simulink library "visionmorphops"  (R2015b)
settings: Solver=ode45  SolverMode=SingleTasking  StartTime=0.0  StopTime=10.0  RelTol=1e-3
undefined symbols (not defined in the file or in its folder): nhdims, nhood
undefined symbols (not defined in the file): strel
libraries: visionmorphops x2
settings Model: ExtModeAutoUpdateStatusClock=off  Creator=The MathWorks, Inc.  LastModifiedBy=The MathWorks, Inc.
settings DataIOCC: SaveFormat=Array  SignalLoggingSaveFormat=ModelDataLogs
settings OptimizationCC: BlockReduction=off  BooleanDataType=off
settings DebuggingCC: SaveWithParameterizedLinksMsg=none  UnderspecifiedInitializationDetection=Classic  MergeDetectMultiDrivingBlocksExec=none  SignalResolutionControl=TryResolveAllWithWarning  StrictBusMsg=Warning
settings HardwareCC: ProdBitPerPointer=32  ProdLargestAtomicFloat=None  ProdIntDivRoundTo=Undefined  ProdEndianess=Unspecified  ProdWordSize=32  ProdHWDeviceType=32-bit Generic  TargetUnknown=on
settings SFSimCC: SimGenImportedTypeDefs=on
settings GRTTargetCC: GeneratePreprocessorConditionals=Disable all
settings ConfigComp: CovModelRefEnable=Off

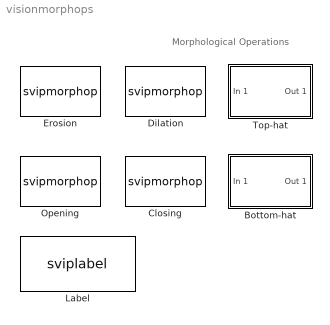
== system visionmorphops ==
  note: Morphological Operations
  Bottom-hat : Subsystem  mask(Bottom-hat){imgtype=Intensity, nhoodsrc=Specify via dialog, strel=strel('octagon',15)}
      mask prompts: imgtype "Input image type:"; nhoodsrc "Neighborhood or structuring element source:"; strel "Neighborhood or structuring element:"
      mask help:
      | Perform morphological bottom-hat filtering on an intensity or binary image.
      |
      | Use the Neighborhood or structuring element parameter to define the neighborhood or structuring element that the block applies to the image.  Specify a neighborhood by entering a matrix or vector of ones and zeros.  Specify a structuring element using the strel function.  Alternatively, you can specify neighborhood values using the Nhood port.
      |
      | For further information on structuring elements, type doc strel at the MATLAB command prompt.
      mask init:
      | nhoodsrc_str = get_param(gcbh,'nhoodsrc');
      | imgtype_str  = get_param(gcbh,'imgtype');
      | if strncmp(nhoodsrc_str,'Specify',5)
      | 	[si(1:2).port] = deal(1,1);
      | 	[si(1:2).txt] = deal('','');
      | else
      | 	[si(1:2).port] = deal(1,2);
      | 	if strncmp(imgtype_str,'Bina',4)
      | 		[si(1:2).txt] = deal('BW','Nhood');
      | 	else
      | 		[si(1:2).txt] = deal('I','Nhood');
      | 	end
      | end
      | 
      | vipblkhatfilter('init')
      mask Help: eval('visionblockhelp');
      mask TypeOptions imgtype: Intensity | Binary
      mask TypeOptions nhoodsrc: Specify via dialog | Input port
      mask Callback nhoodsrc: vipblkhatfilter
      mask Display:
      | disp('Bottom-hat')
      | port_label('input',si(1).port, si(1).txt);
      | port_label('input',si(2).port, si(2).txt);
  Closing : S-Function  FunctionName=svipmorphop  Parameters=3,nhoodsrc,nhood,nhdims  SFunctionDeploymentMode=off  EnableBusSupport=on  mask(Closing){nhoodsrc=Specify via dialog, strel=strel('line',5,45)}
      mask prompts: nhoodsrc "Neighborhood or structuring element source:"; strel "Neighborhood or structuring element:"
      mask help:
      | Perform morphological closing on an intensity or binary image.
      |
      | Use the Neighborhood or structuring element parameter to define the neighborhood or structuring element that the block applies to the image.  Specify a neighborhood by entering a matrix or vector of ones and zeros.  Specify a structuring element using the strel function.  Alternatively, you can specify neighborhood values using the Nhood port.
      |
      | For further information on structuring elements, type doc strel at the MATLAB command prompt.
      mask init:
      | nhoodsrc_str = get_param(gcbh,'nhoodsrc');
      | if strncmp(nhoodsrc_str,'Specify',5)
      | 	[si(1:2).port] = deal(1,1);
      | 	[si(1:2).txt] = deal('','');
      | else
      | 	[si(1:2).port] = deal(1,2);
      | 	[si(1:2).txt] = deal('I','Nhood');
      | end
      | [nhood nhdims] = vipblkmorphop(strel);
      mask Help: eval('visionblockhelp');
      mask TypeOptions nhoodsrc: Specify via dialog | Input port
      mask Callback nhoodsrc: vipblkmorphop
      mask Display:
      | disp('Close');
      | port_label('input',si(1).port, si(1).txt);
      | port_label('input',si(2).port, si(2).txt);
  Dilation : S-Function  FunctionName=svipmorphop  Parameters=1,nhoodsrc,nhood,nhdims  SFunctionDeploymentMode=off  EnableBusSupport=on  mask(Dilation){nhoodsrc=Specify via dialog, strel=[1 1; 1 1]}
      mask prompts: nhoodsrc "Neighborhood or structuring element source:"; strel "Neighborhood or structuring element:"
      mask help:
      | Perform morphological dilation on an intensity or binary image.
      |
      | Use the Neighborhood or structuring element parameter to define the neighborhood or structuring element that the block applies to the image.  Specify a neighborhood by entering a matrix or vector of ones and zeros.  Specify a structuring element using the strel function.  Alternatively, you can specify neighborhood values using the Nhood port.
      |
      | For further information on structuring elements, type doc strel at the MATLAB command prompt.
      mask init: same as visionmorphops/Closing
      mask Help: eval('visionblockhelp');
      mask TypeOptions nhoodsrc: Specify via dialog | Input port
      mask Callback nhoodsrc: vipblkmorphop
      mask Display:
      | disp('Dilate');
      | port_label('input',si(1).port, si(1).txt);
      | port_label('input',si(2).port, si(2).txt);
  Erosion : S-Function  FunctionName=svipmorphop  Parameters=0,nhoodsrc,nhood,nhdims  SFunctionDeploymentMode=off  EnableBusSupport=on  mask(Erosion){nhoodsrc=Specify via dialog, strel=strel('square',4)}
      mask prompts: nhoodsrc "Neighborhood or structuring element source:"; strel "Neighborhood or structuring element:"
      mask help:
      | Perform morphological erosion on an intensity or binary image.
      |
      | Use the Neighborhood or structuring element parameter to define the neighborhood or structuring element that the block applies to the image.  Specify a neighborhood by entering a matrix or vector of ones and zeros.  Specify a structuring element using the strel function.  Alternatively, you can specify neighborhood values using the Nhood port.
      |
      | For further information on structuring elements, type doc strel at the MATLAB command prompt.
      mask init:
      | nhoodsrc_str = get_param(gcbh,'nhoodsrc');
      | if strncmp(nhoodsrc_str,'Specify',5)
      | 	[si(1:2).port] = deal(1,1);
      | 	[si(1:2).txt] = deal('','');
      | else
      | 	[si(1:2).port] = deal(1,2);
      | 	[si(1:2).txt] = deal('I','Nhood');
      | end
      | [nhood nhdims] = vipblkmorphop(strel);
      mask Help: eval('visionblockhelp');
      mask TypeOptions nhoodsrc: Specify via dialog | Input port
      mask Callback nhoodsrc: vipblkmorphop
      mask Display:
      | disp('Erode');
      | port_label('input',si(1).port, si(1).txt);
      | port_label('input',si(2).port, si(2).txt);
  Label : S-Function  FunctionName=sviplabel  Parameters=conn,output,outType,lastLabel  SFunctionDeploymentMode=off  EnableBusSupport=off  mask(Label){conn=8, output=Label matrix and number of labels, outType=Automatic, lastLabel=maximum value of the output data type}
      mask prompts: conn "Connectivity:"; outType "Output data type:"; lastLabel "If label exceeds data type size, mark remaining regions using:"
      mask help:
      | Labels and counts connected components in a binary image.
      |
      | At the Label port, the block outputs a label matrix where pixels equal to 0 represent the background, pixels equal to 1 represent the first object, pixels equal to 2 represent the second object, and so on.  At the Count port, block outputs a scalar that represents the number of labeled objects.
      |
      | Use the Connectivity parameter to define which pixels are connected to each other.
      mask init:
      | output_str = get_param(gcbh,'output');
      | if strncmp(output_str,'Label matrix and',16)
      |     [so(1:2).port] = deal(1,2);
      |     [so(1:2).txt] = deal('Label','Count');
      | elseif strcmp(output_str,'Label matrix')
      |     [so(1:2).port] = deal(1,1);
      |     [so(1:2).txt] = deal('Label','Label');
      | else
      |     [so(1:2).port] = deal(1,1);
      |     [so(1:2).txt] = deal('Count','Count');
      | end
      mask Help: eval('visionblockhelp');
      mask TypeOptions conn: 8 | 4
      mask TypeOptions output: Label matrix and number of labels | Label matrix | Number of labels
      mask TypeOptions outType: Automatic | uint32 | uint16 | uint8
      mask Callback outType: vipblklabel
      mask TypeOptions lastLabel: maximum value of the output data type | zero
      mask Display:
      | disp('Label');
      | port_label('input',1,'BW');
      | port_label('output',so(1).port,so(1).txt);
      | port_label('output',so(2).port,so(2).txt);
  Opening : S-Function  FunctionName=svipmorphop  Parameters=2,nhoodsrc,nhood,nhdims  SFunctionDeploymentMode=off  EnableBusSupport=on  mask(Opening){nhoodsrc=Specify via dialog, strel=strel('disk',5)}
      mask prompts: nhoodsrc "Neighborhood or structuring element source:"; strel "Neighborhood or structuring element:"
      mask help:
      | Perform morphological opening on an intensity or binary image.
      |
      | Use the Neighborhood or structuring element parameter to define the neighborhood or structuring element that the block applies to the image.  Specify a neighborhood by entering a matrix or vector of ones and zeros.  Specify a structuring element using the strel function.  Alternatively, you can specify neighborhood values using the Nhood port.
      |
      | For further information on structuring elements, type doc strel at the MATLAB command prompt.
      mask init: same as visionmorphops/Erosion
      mask Help: eval('visionblockhelp');
      mask TypeOptions nhoodsrc: Specify via dialog | Input port
      mask Callback nhoodsrc: vipblkmorphop
      mask Display:
      | disp('Open');
      | port_label('input',si(1).port, si(1).txt);
      | port_label('input',si(2).port, si(2).txt);
  Top-hat : Subsystem  mask(Top-hat){imgtype=Intensity, nhoodsrc=Specify via dialog, strel=strel('square',4);}
      mask prompts: imgtype "Input image type:"; nhoodsrc "Neighborhood or structuring element source:"; strel "Neighborhood or structuring element:"
      mask help:
      | Perform morphological top-hat filtering on an intensity or binary image.
      |
      | Use the Neighborhood or structuring element parameter to define the neighborhood or structuring element that the block applies to the image.  Specify a neighborhood by entering a matrix or vector of ones and zeros.  Specify a structuring element using the strel function.  Alternatively, you can specify neighborhood values using the Nhood port.
      |
      | For further information on structuring elements, type doc strel at the MATLAB command prompt.
      mask init:
      | nhoodsrc_str = get_param(gcbh,'nhoodsrc');
      | imgtype_str = get_param(gcbh,'imgtype');
      | if strncmp(nhoodsrc_str,'Specify',5)
      | 	[si(1:2).port] = deal(1,1);
      | 	[si(1:2).txt] = deal('','');
      | else
      | 	[si(1:2).port] = deal(1,2);
      | 	if strncmp(imgtype_str,'Bina',4)
      | 		[si(1:2).txt] = deal('BW','Nhood');
      | 	else
      | 		[si(1:2).txt] = deal('I','Nhood');
      | 	end
      | end
      | 
      | vipblkhatfilter('init');
      mask Help: eval('visionblockhelp');
      mask TypeOptions imgtype: Intensity | Binary
      mask TypeOptions nhoodsrc: Specify via dialog | Input port
      mask Callback nhoodsrc: vipblkhatfilter
      mask Display:
      | disp('Top-hat')
      | port_label('input',si(1).port, si(1).txt);
      | port_label('input',si(2).port, si(2).txt);

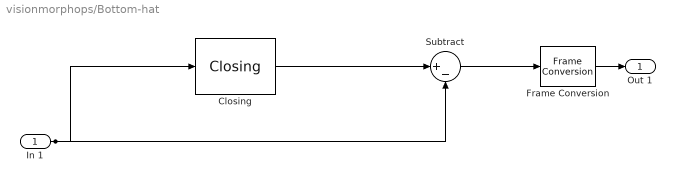
== system visionmorphops/Bottom-hat ==
  In 1 : Inport
  Closing : visionmorphops/Closing  nhoodsrc=Specify via dialog  strel=strel
  Frame Conversion : FrameConversion  InheritSamplingMode=off  OutFrame=Sample-based
  Subtract : Sum  Inputs=|+-  SaturateOnIntegerOverflow=on  InputSameDT=on  OutDataTypeStr=Inherit: Same as first input
  Out 1 : Outport
  wires:
  In 1/1 -> Closing/1, Subtract/2
  Closing/1 -> Subtract/1
  Frame Conversion/1 -> Out 1/1
  Subtract/1 -> Frame Conversion/1

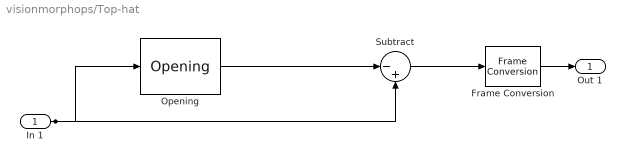
== system visionmorphops/Top-hat ==
  In 1 : Inport
  Frame Conversion : FrameConversion  InheritSamplingMode=off  OutFrame=Sample-based
  Opening : visionmorphops/Opening  nhoodsrc=Specify via dialog  strel=strel
  Subtract : Sum  Inputs=|-+  SaturateOnIntegerOverflow=on  InputSameDT=on  OutDataTypeStr=Inherit: Same as first input
  Out 1 : Outport
  wires:
  In 1/1 -> Opening/1, Subtract/2
  Opening/1 -> Subtract/1
  Subtract/1 -> Frame Conversion/1
  Frame Conversion/1 -> Out 1/1
